simulink model "starshotsim_dev"  (R2023a)
settings: Solver=FixedStepAuto  StartTime=0.0  StopTime=350000  FixedStep=0.01  MaxStep=4.0  MinStep=.001  RelTol=1e-6
values from neighbouring files (symbols this model uses):
  B0 = 3.12e-5    (= 3.12e-05)    [starshot_ACS_setup.m]
  G = 6.67e-11    [starshot_ACS_setup.m]
  M_Earth = 5.972e24    (= 5.972e+24)    [starshot_ACS_setup.m]
  q0 = [qmatlab(2:4),qmatlab(1)]'    [starshot_ACS_setup.m]
  R_Earth = 6.378e6    (= 6378000)    [starshot_ACS_setup.m]
undefined symbols (not defined in the file or in its folder): DiscIntNeverNeededParam, starshot
libraries: simulink x3, dspmathops x3, vrlib x2, sharedtransform x1
(part 2 of 2)

== system starshotsim_dev/StarshotACS/Orientation controller/Subsystem1 ==
  omega : Inport
  B(body) : Inport  Port=2
  Add : Sum  Inputs=3
  Constant3 : Constant
  Constant4 : Constant  Value=-1
  Demux11 : Demux  Outputs=3
  Divide6 : Product  Inputs=/*/
  Norm4 : Subsystem
  Norm5 : Subsystem
  Product3 : Product
  Switch : Switch  Criteria=u2 > Threshold  ZeroCross=off  SaturateOnIntegerOverflow=off  InputSameDT=off
  sign(cos) : Outport
  wires:
  Switch/1 -> sign(cos)/1
  Constant4/1 -> Switch/3
  Add/1 -> Divide6/2
  Constant3/1 -> Switch/1
  Demux11/3 -> Add/3
  Norm4/1(norm(v)) -> Divide6/1
  Divide6/1 -> Switch/2
  Norm5/1(norm(v)) -> Divide6/3
  Product3/1 -> Demux11/1
  Demux11/1 -> Add/1
  Demux11/2 -> Add/2
  B(body)/1 -> Norm5/1(v), Product3/2
  omega/1 -> Product3/1, Norm4/1(v)

== system starshotsim_dev/StarshotACS/Orientation controller/sign_function1 ==
  omega : Inport
  Constant10 : Constant  Value=-1
  Constant9 : Constant
  Selector : Selector  InputPortWidth=3  IndexOptions=Index vector (dialog)  Indices=[3]  OutputSizes=1
  Switch1 : Switch  ZeroCross=off  SaturateOnIntegerOverflow=off  InputSameDT=off
  sign(omega_z) : Outport
  wires:
  Constant9/1 -> Switch1/1
  Constant10/1 -> Switch1/3
  Switch1/1 -> sign(omega_z)/1
  Selector/1 -> Switch1/2
  omega/1 -> Selector/1

== system starshotsim_dev/Plant_OG(Davide's Original)/   /Normalized quat/Modulo1 ==
  q : Inport
  Demux2 : Demux
      settings: DisplayOption=none
  Math Function{1..4} (4 alike) : Math  Operator=square  SignedPower=on
  Math Function5 : Math  Operator=sqrt  SignedPower=on
  Sum5 : Sum  Inputs=|++++  SaturateOnIntegerOverflow=on
  Module q : Outport
  wires:
  q/1 -> Demux2/1
  Math Function5/1 -> Module q/1
  Sum5/1 -> Math Function5/1
  Math Function4/1 -> Sum5/3
  Math Function3/1 -> Sum5/2
  Math Function1/1 -> Sum5/1
  Demux2/3 -> Math Function4/1
  Demux2/2 -> Math Function3/1
  Demux2/1 -> Math Function1/1
  Demux2/4 -> Math Function2/1
  Math Function2/1 -> Sum5/4

== system starshotsim_dev/StarshotACS/Orientation controller/Subsystem1/Norm4 ==
  v : Inport
  Dot Product6 : DotProduct  OutDataTypeStr=Inherit: Inherit via internal rule
  Sqrt4 : Sqrt
  norm(v) : Outport
  wires:
  v/1 -> Dot Product6/1, Dot Product6/2
  Dot Product6/1 -> Sqrt4/1
  Sqrt4/1 -> norm(v)/1

== system starshotsim_dev/StarshotACS/Orientation controller/Subsystem1/Norm5 ==
  v : Inport
  Dot Product6 : DotProduct  OutDataTypeStr=Inherit: Inherit via internal rule
  Sqrt4 : Sqrt
  norm(v) : Outport
  wires:
  v/1 -> Dot Product6/1, Dot Product6/2
  Dot Product6/1 -> Sqrt4/1
  Sqrt4/1 -> norm(v)/1
